simulink model "Buoy_TD_model"  (R2023a)
settings: Solver=VariableStepAuto  StartTime=0.0  StopTime=t(end)  FixedStep=dt  RelTol=1e-3
values from neighbouring files (symbols this model uses):
  Ass = ss2.a    [TD_main.m]    (also in ss_identification.m)
  Bes = 1e4*Bext    [Piston_main_nom.m]    (also in Piston_main_varyT.m; TD_main.m)
  Bext = SF^2.5*Bext_ref    (= 2000)    [Hydrodynamic_parameters_scaling.m]
  Bpto = 0    [Piston_main_nom.m]    (also in Piston_main_varyT.m; TD_main.m)
  Bss = ss2.b    [TD_main.m]    (also in ss_identification.m)
  Css = ss2.c    [TD_main.m]    (also in ss_identification.m)
  d = SF*d_ref    (= 4.7)    [Hydrodynamic_parameters_scaling.m]
  Fw = compute_Fw(ss_type, H, T, omega, gamma, t)    [Piston_main_nom.m]    (also in Piston_main_varyT.m; TD_main.m = Fw + gamma(i)*sqrt(2*(omega(2)-omega(1))*Som(i))*sin(omega(i; compute_Fw.m = Fw + gamma(i)*sqrt(2*(omega(2)-omega(1))*Som(i))*sin(omega(i)
  Kb = rho*g*pi*r^2    (= 198397.46656)    [Hydrodynamic_parameters_scaling.m]
  Kes = 1e0*Kb    [Piston_main_nom.m]    (also in Piston_main_varyT.m; TD_main.m)
  Kpto = 0    [Piston_main_nom.m]    (also in Piston_main_varyT.m; TD_main.m)
  M = SF^3*M_ref    [Hydrodynamic_parameters_scaling.m]
  Vmax = 20    [Piston_main_nom.m]    (also in Piston_main_varyT.m; TD_main.m)
settings Model: Creator=Unitn  LastModifiedBy=Unitn
settings DataIOCC: ReturnWorkspaceOutputs=off

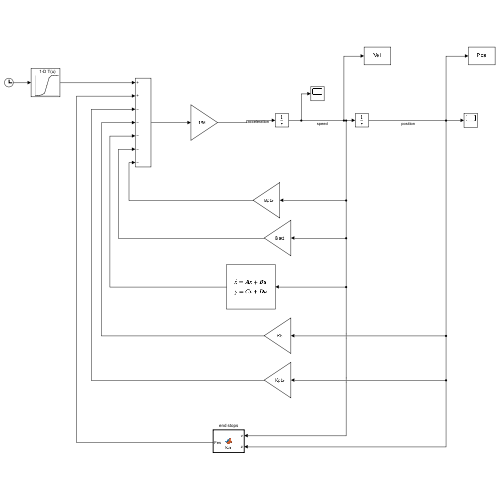
[thumbnail: Simulink's stored preview of the top-level diagram]
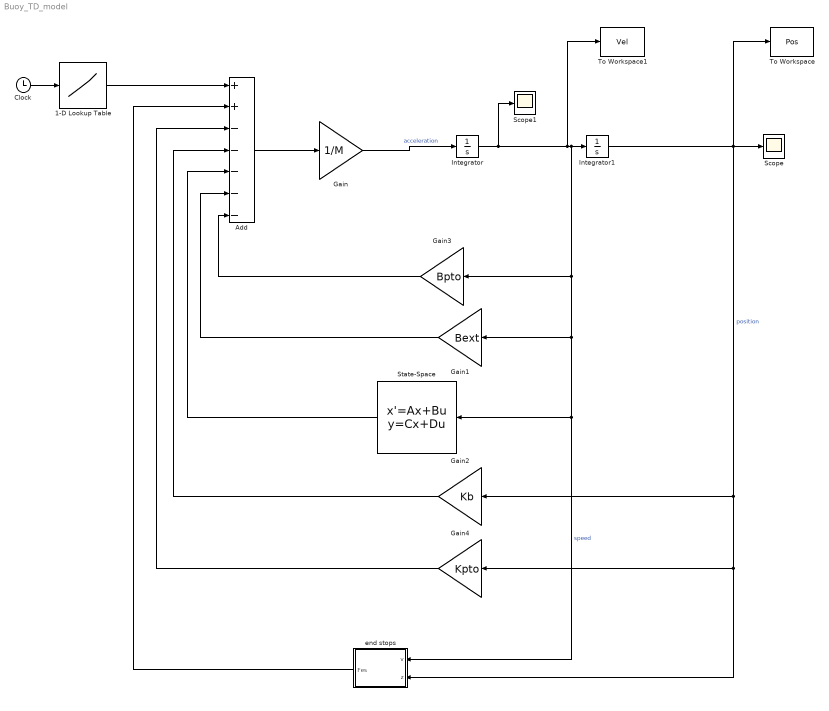
== system Buoy_TD_model ==
  1-D Lookup Table : Lookup_n-D  NumberOfTableDimensions=1  BreakpointsForDimension1=t  Table=Fw  InternalRulePriority=Speed  RndMeth=Simplest
  Add : Sum  Inputs=++-----
  Clock : Clock
  Gain : Gain  Gain=1/M
  Gain1 : Gain  Gain=Bext
  Gain2 : Gain  Gain=Kb
  Gain3 : Gain  Gain=Bpto
  Gain4 : Gain  Gain=Kpto
  Integrator : Integrator
  Integrator1 : Integrator
  Scope : Scope
  Scope1 : Scope
  State-Space : StateSpace  A=Ass  B=Bss  C=Css  D=0  InitialCondition=0
  To Workspace : ToWorkspace  VariableName=Pos  SaveFormat=Timeseries  SampleTime=-1
  To Workspace1 : ToWorkspace  VariableName=Vel  SaveFormat=Timeseries  SampleTime=-1
  end stops : MATLAB Function  TreatAsAtomicUnit=on
  wires:
  Add/1 -> Gain/1
  Gain/1 -> Integrator/1  "acceleration"
  Integrator/1 -> Scope1/1, Gain3/1, end stops/1(v), State-Space/1, Gain1/1, Integrator1/1, To Workspace1/1  "speed"
  Integrator1/1 -> To Workspace/1, end stops/2(z), Gain4/1, Gain2/1, Scope/1  "position"
  Gain1/1 -> Add/6
  Gain2/1 -> Add/4
  Clock/1 -> 1-D Lookup Table/1
  1-D Lookup Table/1 -> Add/1
  State-Space/1 -> Add/5
  Gain3/1 -> Add/7
  Gain4/1 -> Add/3
  end stops/1(Fes) -> Add/2

== matlab function Buoy_TD_model/end stops ==
  data: v input; Fes output; z input; d parameter; Kes parameter; Bes parameter; Vmax parameter
function Fes = fcn(v,z,d,Kes, Bes, Vmax)

if abs(z)<d
    Fes = 0;
elseif z>d
    Fes = -Kes*(z-d)-Bes*v;
else
    Fes = -Kes*(z+d)-Bes*v;
end

if abs(v)>Vmax
    Fes = Fes -Bes*v;
end
